simulink model "Eq_Zeq_total"  (R2022a)
settings: Solver=VariableStepAuto  StartTime=0.0  StopTime=10.0  RelTol=1e-3
libraries: cstblocks x1
settings Model: Creator=umber  LastModifiedBy=umber

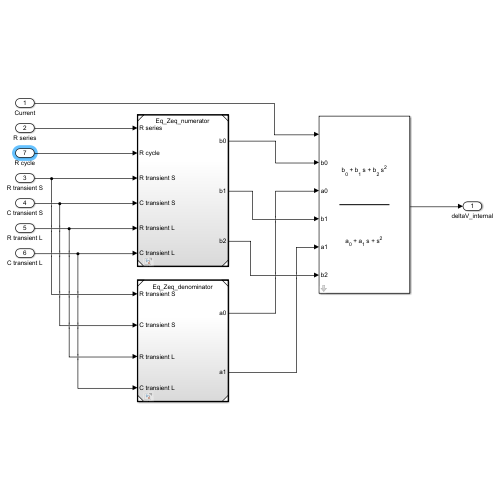
[thumbnail: Simulink's stored preview of the top-level diagram]
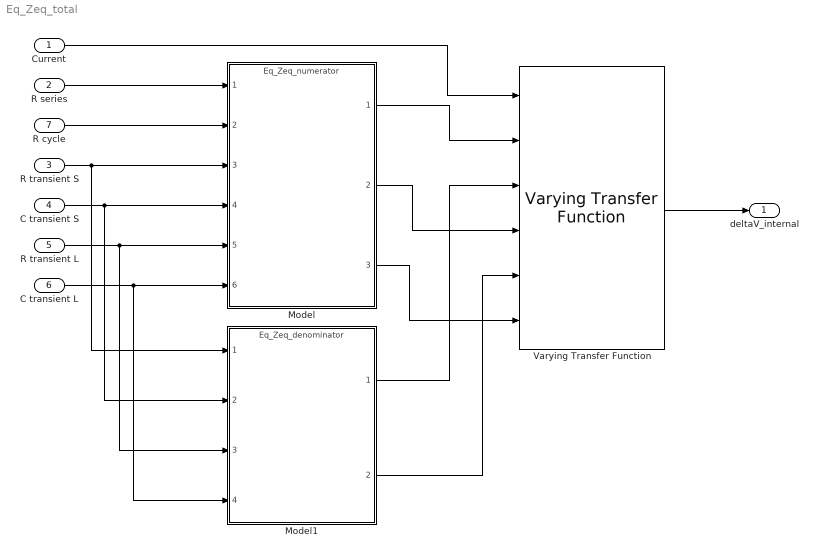
== system Eq_Zeq_total ==
  Current : Inport
  R series : Inport  Port=2
  R transient S : Inport  Port=3
  C transient S : Inport  Port=4
  R transient L : Inport  Port=5
  C transient L : Inport  Port=6
  R cycle : Inport  Port=7
  Model : ModelReference  ModelNameDialog=Eq_Zeq_numerator.slx  SimulationMode=Normal  ModelReferenceVersion=1.1
  Model1 : ModelReference  ModelNameDialog=Eq_Zeq_denominator.slx  SimulationMode=Normal  ModelReferenceVersion=1.3
  Varying Transfer Function : cstblocks/Linear Parameter Varying/Varying Transfer Function  N=2
  deltaV_internal : Outport
  wires:
  R series/1 -> Model/1
  R cycle/1 -> Model/2
  R transient S/1 -> Model1/1, Model/3
  C transient S/1 -> Model1/2, Model/4
  R transient L/1 -> Model1/3, Model/5
  C transient L/1 -> Model1/4, Model/6
  Model1/1 -> Varying Transfer Function/3
  Model1/2 -> Varying Transfer Function/5
  Model/3 -> Varying Transfer Function/6
  Model/2 -> Varying Transfer Function/4
  Model/1 -> Varying Transfer Function/2
  Current/1 -> Varying Transfer Function/1
  Varying Transfer Function/1 -> deltaV_internal/1
